simulink model "qep_calibration_host"  (R2025b)
settings: Solver=FixedStepDiscrete  StartTime=0.0  StopTime=Inf  RelTol=1e-3
undefined symbols (not defined in the file or in its folder): motor
libraries: instrumentseriallib x3, simulink x1

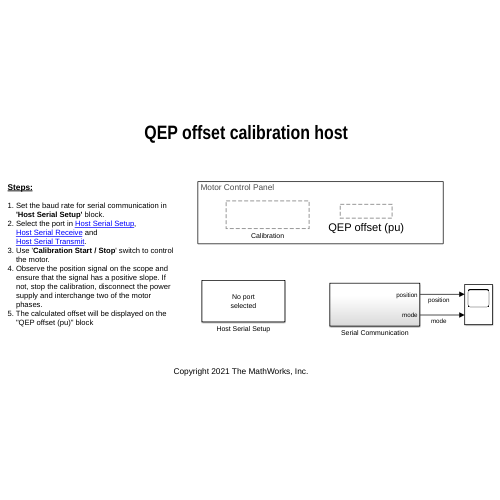
[thumbnail: Simulink's stored preview of the top-level diagram]
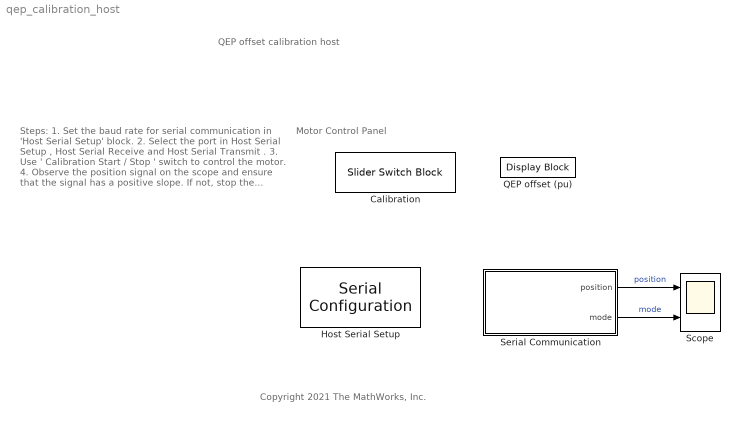
== system qep_calibration_host ==
  note: QEP offset calibration host
  note: Motor Control Panel
  note: Steps:
      |
      | 1. Set the baud rate for serial communication in
      | 'Host Serial Setup' block.
      | 2. Select the port in Host Serial Setup ,
      | Host Serial Receive and
      | Host Serial Transmit .
      | 3. Use ' Calibration Start / Stop ' switch to control
      | the motor.
      | 4. Observe the position signal on the scope and
      | ensure that the signal has a positive slope. If
      | not, stop the calibration, disconnect the power
      | supply and interchange two of the motor
      | phases.
      | 5. The calculated offset will be displayed on the
      | "QEP offset (pu)" block
  note: Copyright 2021 The MathWorks, Inc.
  Calibration : SliderSwitchBlock  LabelPosition=Hide
  Host Serial Setup : instrumentseriallib/Serial Configuration  Priority=-99  PortSel=<Select a port...>  Port=<Select a port...>  ComPort=<Select a port...>  BaudRate=4000000  DataBits=8  Parity=none  StopBits=1  ByteOrder=little-endian  FlowControl=none  Timeout=2.0  SimulateUsing=Interpreted execution  BlockInModel=on  aMode=5
  QEP offset (pu) : DisplayBlock  LabelPosition=Hide  Transparency=1  GridColor=[0.502, 0.502, 0.502]
  Scope : Scope  NumInputPorts=2
  Serial Communication : Subsystem
  wires:
  Serial Communication/1(position) -> Scope/1  "position"
  Serial Communication/2(mode) -> Scope/2  "mode"

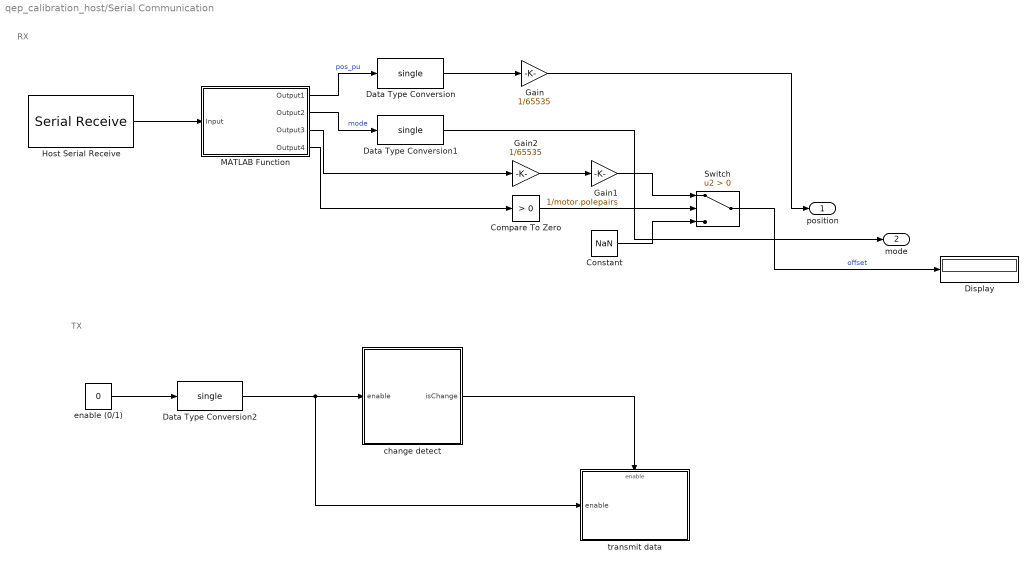
== system qep_calibration_host/Serial Communication ==
  note: TX
  note: RX
  Compare To Zero : simulink/Logic and Bit Operations/Compare To Zero  relop=>  OutDataTypeStr=boolean
  Constant : Constant  Value=NaN  OutDataTypeStr=single
  Data Type Conversion : DataTypeConversion  OutDataTypeStr=single  SaturateOnIntegerOverflow=off  RndMeth=Floor
  Data Type Conversion1 : DataTypeConversion  OutDataTypeStr=single  SaturateOnIntegerOverflow=off  RndMeth=Floor
  Data Type Conversion2 : DataTypeConversion  OutDataTypeStr=single  SaturateOnIntegerOverflow=off  RndMeth=Floor
  Display : Display
  Gain : Gain  Gain=1/65535  OutDataTypeStr=single
  Gain1 : Gain  Gain=1/motor.polepairs  OutDataTypeStr=single
  Gain2 : Gain  Gain=1/65535  OutDataTypeStr=single
  Host Serial Receive : instrumentseriallib/Serial Receive  PortSel=<Select a port...>  Port=<Select a port...>  ComPort=<Select a port...>  DataType=uint16  SaveDataType=uint8  ToggleHeader=on  Header='ss'  ToggleDataSize=on  DataSize=[200 2]  ToggleTerminator=on  Terminator=Custom terminator  CustomTerminator='ee'  InputFormat=Row major  EnableBlockingMode=on  ActionDataUnavailable=Output custom value  ActionWhenDataUnavailable=Output custom value  CustomValue=4000  SampleTime=200 * 50e-6  SimulateUsing=Interpreted execution  BlockInModel=on  aMode=5  LibraryInUse=instrumentlib
  MATLAB Function : MATLAB Function  TreatAsAtomicUnit=on
  Switch : Switch  Criteria=u2 > Threshold  SaturateOnIntegerOverflow=off  InputSameDT=off
  change detect : Subsystem
  enable (0/1) : Constant  Value=0  OutDataTypeStr=boolean  SampleTime=-1
  transmit data : Subsystem  TreatAsAtomicUnit=on
  position : Outport
  mode : Outport  Port=2
  wires:
  Gain/1 -> position/1
  Data Type Conversion1/1 -> mode/1
  Switch/1 -> Display/1  "offset"
  Data Type Conversion/1 -> Gain/1
  Gain1/1 -> Switch/1
  MATLAB Function/2(Output2) -> Data Type Conversion1/1  "mode"
  Compare To Zero/1 -> Switch/2
  MATLAB Function/3(Output3) -> Gain2/1
  MATLAB Function/4(Output4) -> Compare To Zero/1
  Gain2/1 -> Gain1/1
  Host Serial Receive/1 -> MATLAB Function/1(Input)
  Constant/1 -> Switch/3
  MATLAB Function/1(Output1) -> Data Type Conversion/1  "pos_pu"
  Data Type Conversion2/1 -> transmit data/1(enable), change detect/1(enable)
  change detect/1(isChange) -> transmit data/Enable
  enable (0/1)/1 -> Data Type Conversion2/1

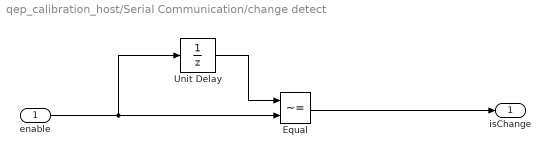
== system qep_calibration_host/Serial Communication/change detect ==
  enable : Inport
  Equal : RelationalOperator  Operator=~=  OutDataTypeStr=boolean  RndMeth=Simplest  InputSameDT=off
  Unit Delay : UnitDelay  SampleTime=-1  HasFrameUpgradeWarning=on
  isChange : Outport
  wires:
  Unit Delay/1 -> Equal/1
  enable/1 -> Equal/2, Unit Delay/1
  Equal/1 -> isChange/1

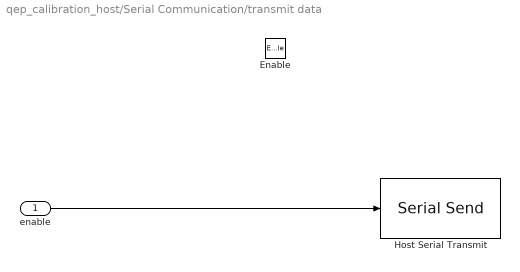
== system qep_calibration_host/Serial Communication/transmit data ==
  enable : Inport
  Enable : EnablePort
  Host Serial Transmit : instrumentseriallib/Serial Send  PortSel=<Select a port...>  Port=<Select a port...>  ComPort=<Select a port...>  Header=[]  Terminator=<none>  CustomTerminator=[]  EnableBlockingMode=off  SimulateUsing=Interpreted execution  BlockInModel=on  aMode=5
  wires:
  enable/1 -> Host Serial Transmit/1

== matlab function qep_calibration_host/Serial Communication/MATLAB Function ==
function [Output1, Output2, Output3, Output4]  = unBuf(Input)

Output1 = Input(:, 1);
Output2 = Input(:, 2);
Output3 = Output1(1);
Output4 = Output2(1);

end
